simulink model "Rotor_flux_observer_with_arbitrary_rate_of_convergence"  (R2021a)
settings: Solver=VariableStepAuto  StartTime=0.0  StopTime=10.0  RelTol=1e-3
settings Model: Creator=Mehra  LastModifiedBy=Mehra

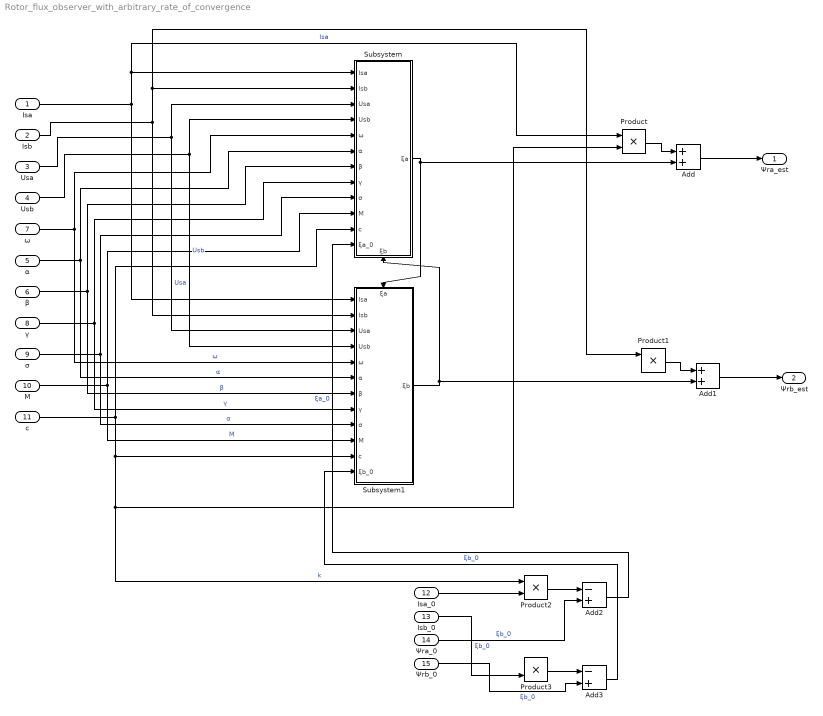
== system Rotor_flux_observer_with_arbitrary_rate_of_convergence ==
  Isa : Inport
  Isb : Inport  Port=2
  Usa : Inport  Port=3
  Usb : Inport  Port=4
  α : Inport  Port=5
  β : Inport  Port=6
  ω : Inport  Port=7
  γ : Inport  Port=8
  σ : Inport  Port=9
  M : Inport  Port=10
  c : Inport  Port=11
  Isa_0 : Inport  Port=12
  Isb_0 : Inport  Port=13
  Ψra_0 : Inport  Port=14
  Ψrb_0 : Inport  Port=15
  Add : Sum
  Add1 : Sum
  Add2 : Sum  Inputs=-+
  Add3 : Sum  Inputs=-+
  Product{,1..3} (4 alike) : Product
  Subsystem : Subsystem
      settings: PortSchema="{\"entries\":[{\"content\":{\"sides\":[{\"content\":{\"connectorIds\":[\"In1\",\"In2\",\"In3\",\"In4\",\"In5\",\"In6\",\"In7\",\"In8\",\"In9\",\"In10\",\"In11\",\"In12\"]},\"type\":\"ConnectorPlacement.EquallySpacedRectSide\",\"uuid\":\"d464ab2a-d91e-4fa3-84c4-bb548725a2b5\"},{\"content\":{\"connectorIds\":[\"Out1\"],\"side\":\"RIGHT\"},\"type\":\"ConnectorPlacement.EquallySpacedRectSide\",\"uuid\":\"bbde90e7-174a-4034-b09b-29d4ce63dbf9\"},{\"content\":{\"connectorIds\":[],\"side\":\"TOP\"},\"type\":\"ConnectorPlacement.EquallySpacedRectSide\",\"uuid\":\"6d5817a3-48e6-4f2f-a59d-d9d2dfa8c415\"},{\"content\":{\"connectorIds\":[\"In13\"],\"side\":\"BOTTOM\"},\"type\":\"ConnectorPlacement.EquallySpacedRectSide\",\"uuid\":\"1f70f23a-d63b-4e2d-b056-8428cf1e3bc1\"}]},\"type\":\"ConnectorPlacement.EquallySpacedConnector\",\"uuid\":\"0f767fdf-fe9d-47e8-b76d-bfc140dd9a1b\"}],\"packageUris\":[\"http://schema.mathworks.com/mf0/Connector/R2020b\"],\"version\":\"1.0\"}"
  Subsystem1 : Subsystem
      settings: PortSchema="{\"entries\":[{\"content\":{\"sides\":[{\"content\":{\"connectorIds\":[\"In1\",\"In2\",\"In3\",\"In4\",\"In5\",\"In6\",\"In7\",\"In8\",\"In9\",\"In10\",\"In11\",\"In12\"]},\"type\":\"ConnectorPlacement.EquallySpacedRectSide\",\"uuid\":\"d464ab2a-d91e-4fa3-84c4-bb548725a2b5\"},{\"content\":{\"connectorIds\":[\"Out1\"],\"side\":\"RIGHT\"},\"type\":\"ConnectorPlacement.EquallySpacedRectSide\",\"uuid\":\"bbde90e7-174a-4034-b09b-29d4ce63dbf9\"},{\"content\":{\"connectorIds\":[\"In13\"],\"side\":\"TOP\"},\"type\":\"ConnectorPlacement.EquallySpacedRectSide\",\"uuid\":\"6d5817a3-48e6-4f2f-a59d-d9d2dfa8c415\"}]},\"type\":\"ConnectorPlacement.EquallySpacedConnector\",\"uuid\":\"0f767fdf-fe9d-47e8-b76d-bfc140dd9a1b\"}],\"packageUris\":[\"http://schema.mathworks.com/mf0/Connector/R2020b\"],\"version\":\"1.0\"}"
  Ψra_est : Outport
  Ψrb_est : Outport  Port=2
  wires:
  Isa/1 -> Subsystem1/1(Isa), Product/1, Subsystem/1(Isa)  "Isa"
  Isb/1 -> Product1/1, Subsystem/2(Isb), Subsystem1/2(Isb)
  Usa/1 -> Subsystem1/3(Usa), Subsystem/3(Usa)  "Usa"
  Usb/1 -> Subsystem1/4(Usb), Subsystem/4(Usb)  "Usb"
  ω/1 -> Subsystem1/5(ω), Subsystem/5(ω)  "ω"
  α/1 -> Subsystem1/6(α), Subsystem/6(α)  "α"
  β/1 -> Subsystem1/7(β), Subsystem/7(β)  "β"
  γ/1 -> Subsystem1/8(γ), Subsystem/8(γ)  "γ"
  σ/1 -> Subsystem1/9(σ), Subsystem/9(σ)  "σ"
  M/1 -> Subsystem1/10(M), Subsystem/10(M)  "M"
  c/1 -> Product/2, Product2/1, Subsystem1/11(c), Subsystem/11(c)  "k"
  Subsystem1/1(ξb) -> Subsystem/13(ξb), Add1/2
  Subsystem/1(ξa) -> Subsystem1/13(ξa), Add/2
  Product/1 -> Add/1
  Add/1 -> Ψra_est/1
  Product1/1 -> Add1/1
  Add1/1 -> Ψrb_est/1
  Isa_0/1 -> Product2/2
  Product2/1 -> Add2/1
  Ψra_0/1 -> Add2/2  "ξb_0"
  Isb_0/1 -> Product3/2  "ξb_0"
  Product3/1 -> Add3/1
  Ψrb_0/1 -> Add3/2  "ξb_0"
  Add2/1 -> Subsystem/12(ξa_0)  "ξa_0"
  Add3/1 -> Subsystem1/12(ξb_0)  "ξb_0"

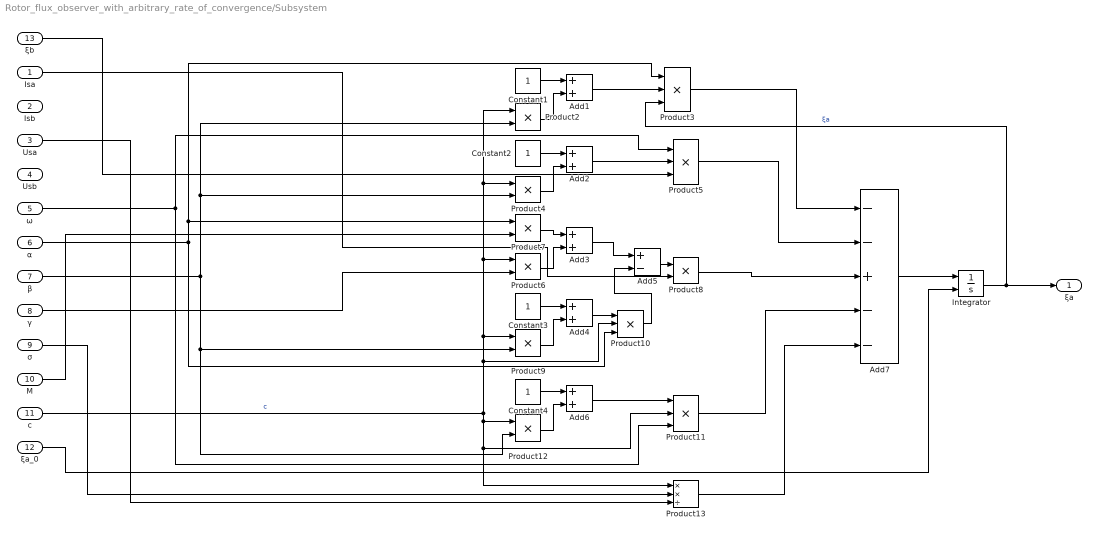
== system Rotor_flux_observer_with_arbitrary_rate_of_convergence/Subsystem ==
  Isa : Inport
  Isb : Inport  Port=2
  Usa : Inport  Port=3
  Usb : Inport  Port=4
  ω : Inport  Port=5
  α : Inport  Port=6
  β : Inport  Port=7
  γ : Inport  Port=8
  σ : Inport  Port=9
  M : Inport  Port=10
  c : Inport  Port=11
  ξa_0 : Inport  Port=12
  ξb : Inport  Port=13
  Add{1..4,6} (5 alike) : Sum
  Add5 : Sum  Inputs=+-
  Add7 : Sum  Inputs=--+--
  Constant{1..4} (4 alike) : Constant
  Integrator : Integrator  InitialConditionSource=external
  Product{3,5,10..11} (4 alike) : Product  Inputs=3
  Product{2,4,6..9,12} (7 alike) : Product
  Product13 : Product  Inputs=**/
  ξa : Outport
  wires:
  Add5/1 -> Product8/1
  σ/1 -> Product13/2
  c/1 -> Product9/1, Product6/1, Product2/1, Product4/1, Product10/2, Product13/1, Product11/2, Product12/1  "c"
  β/1 -> Product4/2, Product2/2, Product9/2, Product12/2
  Add7/1 -> Integrator/1
  α/1 -> Product10/3, Product3/1, Product7/1
  ω/1 -> Product11/3, Product5/1
  γ/1 -> Product6/2
  Product7/1 -> Add3/1
  Product8/1 -> Add7/3
  Product4/1 -> Add2/2
  Constant2/1 -> Add2/1
  Product10/1 -> Add5/2
  Product13/1 -> Add7/5
  Product5/1 -> Add7/2
  Constant4/1 -> Add6/1
  Add2/1 -> Product5/2
  Constant3/1 -> Add4/1
  Product12/1 -> Add6/2
  Integrator/1 -> ξa/1, Product3/3  "ξa"
  ξa_0/1 -> Integrator/2
  Product6/1 -> Add3/2
  Product9/1 -> Add4/2
  ξb/1 -> Product5/3
  Add4/1 -> Product10/1
  Add1/1 -> Product3/2
  Product11/1 -> Add7/4
  Product3/1 -> Add7/1
  Product2/1 -> Add1/2
  Constant1/1 -> Add1/1
  Add3/1 -> Add5/1
  Usa/1 -> Product13/3
  Add6/1 -> Product11/1
  Isa/1 -> Product8/2
  M/1 -> Product7/2

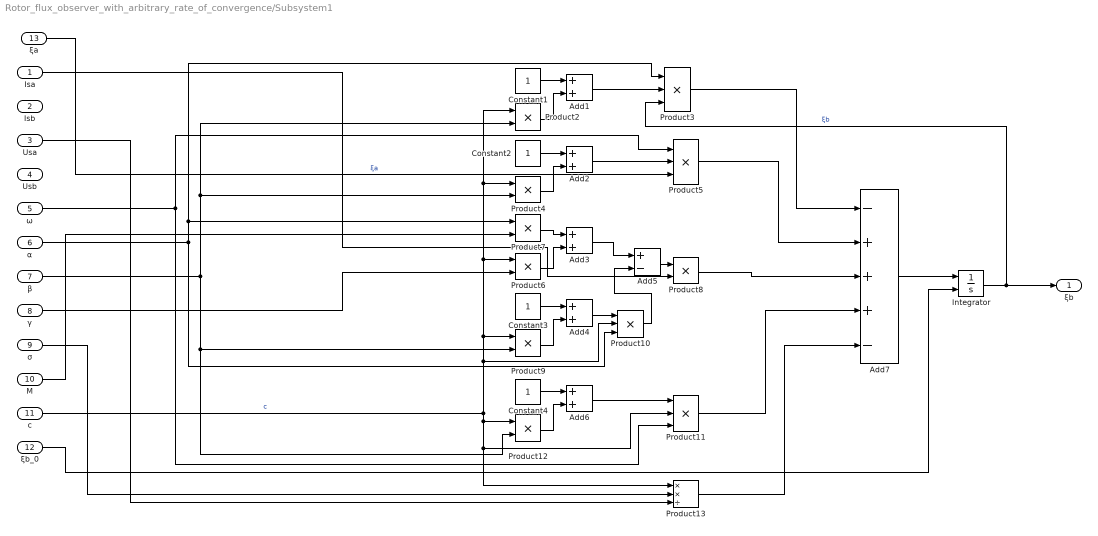
== system Rotor_flux_observer_with_arbitrary_rate_of_convergence/Subsystem1 ==
  Isa : Inport
  Isb : Inport  Port=2
  Usa : Inport  Port=3
  Usb : Inport  Port=4
  ω : Inport  Port=5
  α : Inport  Port=6
  β : Inport  Port=7
  γ : Inport  Port=8
  σ : Inport  Port=9
  M : Inport  Port=10
  c : Inport  Port=11
  ξb_0 : Inport  Port=12
  ξa : Inport  Port=13
  Add{1..4,6} (5 alike) : Sum
  Add5 : Sum  Inputs=+-
  Add7 : Sum  Inputs=-+++-
  Constant{1..4} (4 alike) : Constant
  Integrator : Integrator  InitialConditionSource=external
  Product{3,5,10..11} (4 alike) : Product  Inputs=3
  Product{2,4,6..9,12} (7 alike) : Product
  Product13 : Product  Inputs=**/
  ξb : Outport
  wires:
  Add5/1 -> Product8/1
  σ/1 -> Product13/2
  c/1 -> Product9/1, Product6/1, Product2/1, Product4/1, Product10/2, Product13/1, Product11/2, Product12/1  "c"
  β/1 -> Product4/2, Product2/2, Product9/2, Product12/2
  Add7/1 -> Integrator/1
  α/1 -> Product10/3, Product3/1, Product7/1
  ω/1 -> Product11/3, Product5/1
  γ/1 -> Product6/2
  Product7/1 -> Add3/1
  Product8/1 -> Add7/3
  Product4/1 -> Add2/2
  Constant2/1 -> Add2/1
  Product10/1 -> Add5/2
  Product13/1 -> Add7/5
  Product5/1 -> Add7/2
  Constant4/1 -> Add6/1
  Add2/1 -> Product5/2
  Constant3/1 -> Add4/1
  Product12/1 -> Add6/2
  Integrator/1 -> ξb/1, Product3/3  "ξb"
  ξb_0/1 -> Integrator/2
  Product6/1 -> Add3/2
  Product9/1 -> Add4/2
  ξa/1 -> Product5/3  "ξa"
  Add4/1 -> Product10/1
  Add1/1 -> Product3/2
  Product11/1 -> Add7/4
  Product3/1 -> Add7/1
  Product2/1 -> Add1/2
  Constant1/1 -> Add1/1
  Add3/1 -> Add5/1
  Usa/1 -> Product13/3
  Add6/1 -> Product11/1
  Isa/1 -> Product8/2
  M/1 -> Product7/2
